simulink model "distance_calc"  (Simulink 7.8)
settings: Solver=ode45  StartTime=0.0  StopTime=50.0  RelTol=1e-3
undefined symbols (not defined in the file): gray, none, videoinput
libraries: visionsinks x5, imaqlib x1
settings Model: Creator=wildcat  LastModifiedBy=wildcat

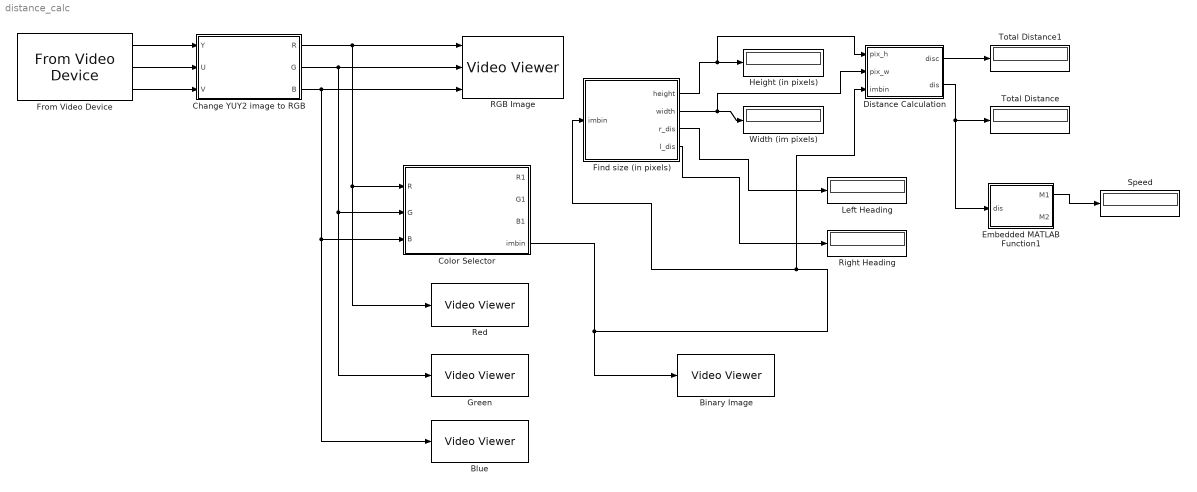
== system distance_calc ==
  Binary Image : visionsinks/Video Viewer  inputType=Obsolete7b  imagePorts=One multidimensional signal  useColorMap=off  colormapValue=gray(256)  specRange=off  minInputVal=0  maxInputVal=255  FigPos=[112 381 430 251]  AxisZoom=on  trueSizedOnce=off  OpenAtMdlStart=on
  Blue : visionsinks/Video Viewer  inputType=Obsolete7b  imagePorts=One multidimensional signal  useColorMap=off  colormapValue=gray(256)  specRange=off  minInputVal=0  maxInputVal=255  FigPos=[42 561 423 342]  AxisZoom=on  trueSizedOnce=off  OpenAtMdlStart=on
  Change YUY2 image to RGB : MATLAB Function  TreatAsAtomicUnit=on
  Color Selector : MATLAB Function  TreatAsAtomicUnit=on
  Distance Calculation : MATLAB Function  TreatAsAtomicUnit=on
  Embedded MATLAB Function1 : MATLAB Function  TreatAsAtomicUnit=on
  Find size (in pixels) : MATLAB Function  TreatAsAtomicUnit=on
  From Video Device : imaqlib/From Video Device  DeviceMenu=winvideo 1 (Microsoft LifeCam HD-3000)  Device=winvideo 1 (Microsoft LifeCam HD-3000)  ObjConstructor=videoinput('winvideo', 1)  VideoFormatMenu=YUY2_1280x720  VideoFormat=YUY2_640x360  VideoSource=input1  ROIPosition=[0 0 360 640]  EnableHWTrigger=off  TriggerConfiguration=none/none  SampleTime=1/30  OutputPortsMode=Separate color signals  DataType=uint8  CanDoHWTrigger=no  ReturnedColorSpace=YCbCr  BlockHandle=77.0012  ROIWidth=640  ROIHeight=360  ROIColumn=0  ROIRow=0  EngXMLPath=C:\Program Files\MatlabR2011b\toolbox\imaq\imaq\private  DevXMLPath=C:\Program Files\MatlabR2011b\toolbox\imaq\imaqadaptors\win64  EngLibPath=C:\Program Files\MatlabR2011b\toolbox\imaq\imaqblks\imaqmex\win64
  Green : visionsinks/Video Viewer  inputType=Obsolete7b  imagePorts=One multidimensional signal  useColorMap=off  colormapValue=gray(256)  specRange=off  minInputVal=0  maxInputVal=255  FigPos=[489 563 423 342]  AxisZoom=on  trueSizedOnce=off  OpenAtMdlStart=on
  Height (in pixels) : Display
  Left Heading : Display
  RGB Image : visionsinks/Video Viewer  inputType=Obsolete7b  imagePorts=Separate color signals  useColorMap=off  colormapValue=gray(256)  specRange=off  minInputVal=0  maxInputVal=255  FigPos=[84 648 822 453]  AxisZoom=on  trueSizedOnce=off  OpenAtMdlStart=on
  Red : visionsinks/Video Viewer  inputType=Obsolete7b  imagePorts=One multidimensional signal  useColorMap=off  colormapValue=gray(256)  specRange=off  minInputVal=0  maxInputVal=255  FigPos=[917 555 423 342]  AxisZoom=on  trueSizedOnce=off  OpenAtMdlStart=on
  Right Heading : Display
  Speed : Display
  Total Distance : Display
  Total Distance1 : Display
  Width (im pixels) : Display
  wires:
  From Video Device/1 -> Change YUY2 image to RGB/1(Y)
  From Video Device/2 -> Change YUY2 image to RGB/2(U)
  From Video Device/3 -> Change YUY2 image to RGB/3(V)
  Change YUY2 image to RGB/3(B) -> RGB Image/3, Color Selector/3(B), Blue/1
  Change YUY2 image to RGB/2(G) -> RGB Image/2, Color Selector/2(G), Green/1
  Change YUY2 image to RGB/1(R) -> RGB Image/1, Color Selector/1(R), Red/1
  Color Selector/4(imbin) -> Binary Image/1, Find size (in pixels)/1(imbin), Distance Calculation/3(imbin)
  Find size (in pixels)/1(height) -> Height (in pixels)/1, Distance Calculation/1(pix_h)
  Find size (in pixels)/2(width) -> Width (im pixels)/1, Distance Calculation/2(pix_w)
  Distance Calculation/2(dis) -> Total Distance/1, Embedded MATLAB Function1/1(dis)
  Find size (in pixels)/3(r_dis) -> Left Heading/1
  Find size (in pixels)/4(l_dis) -> Right Heading/1
  Distance Calculation/1(disc) -> Total Distance1/1
  Embedded MATLAB Function1/1(M1) -> Speed/1

== matlab function Change YUY2 image to RGB ==
  data: Y input double; R output double; G output double; B output double; U input double; V input double
function [R,G,B] = YUY2toRGB(Y,U,V)
%% input is (:,:,1:3), where
%% (:,:,1) is Y, (:,:,2) is U, (:,:,3) is V


%Y = single(data(:,:,1));
%U = single(data(:,:,2));
%V = single(data(:,:,3));

B = 1.164*(Y - 16) + 2.018*(U - 128);

G = 1.164*(Y - 16) - 0.813*(V - 128) - 0.391*(U - 128);

R = 1.164*(Y - 16) + 1.596*(V - 128);

R=uint8(R);
G=uint8(G);
B=uint8(B);

== matlab function Color Selector ==
  data: R input double; R1 output double; G input double; B input double; G1 output double; B1 output double; imbin output double
function [R1,G1,B1,imbin] = color_selection(R,G,B)

imsize = size(R);
imsize = size(G);
imsize = size(B);

R1 = zeros(imsize);
G1 = zeros(imsize);
B1 = zeros(imsize);
imbin = zeros(imsize);

for (imh = 1:imsize(1,1));
    for (iml = 1:imsize(1,2));
        imR = R(imh,iml);
        imG = G(imh,iml);
        imB = B(imh,iml);
        if (imR >= 170) && (imR <= 255) && (imG >= 15) && (imG <= 70) && (imB >= 70) && (imB <= 130)
            R1(imh,iml) = 255;
            G1(imh,iml) = 255;
            B1(imh,iml) = 255;
            imbin(imh,iml) = 1;
        end
    end
end

== matlab function Find size (in pixels) ==
  data: imbin input double; height output double; width output double; r_dis output double; l_dis output double
function [height,width,r_dis,l_dis] = hw_find(imbin)

imsize=size(imbin);

height = 0;
width = 0;
height_sum = 0;
width_sum = 0;
marker = 0;
obstart = 0;

for (imh = 1:imsize(1,1));
    width_sum = 0;
    for (iml = 1:imsize(1,2));
        imloc = imbin(imh,iml);
        if (imloc == 1)
            width_sum=width_sum+1;
        end
    end
    if (width_sum >= 6)
        height = height+1;
    end
end



for (iml = 1:imsize(1,2));
    height_sum = 0;
    for (imh = 1:imsize(1,1));
        imloc = imbin(imh,iml);
        if (imloc == 1)
            height_sum=height_sum+1;
        end
    end
    if (height_sum >= 6)
        width = width+1;
        if (marker == 0)
            marker = 1;
            obstart = iml;
        end
    end
end

obend = obstart + width;

r_dis = obstart;
l_dis = imsize(1,2) - obend;

== matlab function Distance Calculation ==
  data: disc output double; pix_h input double; dis output double; pix_w input double; imbin input double
function [disc,dis] = find_dis(pix_h,pix_w,imbin)

%1.4=2*tan(44.443*pi/360)*dis*height1/480;
%ob_w=2*tan(57.154*pi/360)*dis*width1/640;

imsize = size(imbin);

dis1 = (5.875*imsize(1,1))/(2*tan(44.443*pi/360)*pix_h);

dis2 = (5.5*imsize(1,2))/(2*tan(57.154*pi/360)*pix_w);

dis=(dis1+dis2)/2;

disc = dis*(1-(0.001*dis^2+0.0831*dis-9.4421)/100);

== matlab function Embedded MATLAB Function1 ==
  data: dis input double; M1 output double; M2 output double
function [M1,M2]= fcn(dis)

%Sample speed
M1 = 620-5*dis;
M2 = 620-5*dis;


%Prevent rpm of M1 and M2 from going above 620 or below -620
if (M1 >= 620)
    M1 = 620;
elseif (M1<= -620)
    M2 = -620;
else
    M1 = M1;
end


if (M2 >= 620)
    M2 = 620;
elseif (M2<= -620)
    M2 = -620;
else
    M2 = M2;
end
